simulink model "detection_algorithm_model"  (Simulink 7.7)
settings: Solver=VariableStepDiscrete  StartTime=0.0  StopTime=0.1  RelTol=1e-3
libraries: dsparch4 x1, dspstat3 x1, dspsrcs4 x1
settings Model: Creator=staticd  LastModifiedBy=staticd

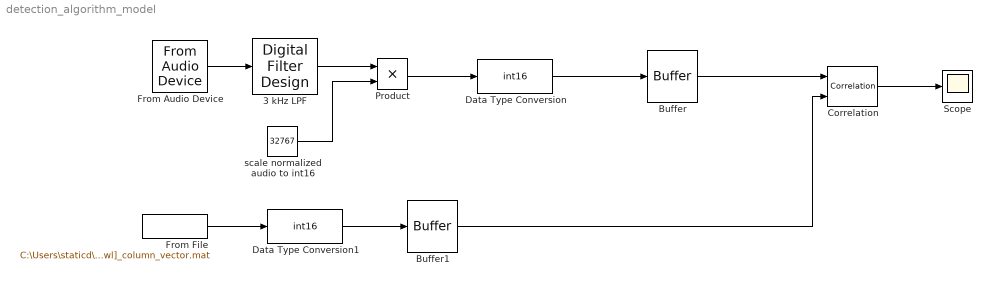
== system detection_algorithm_model ==
  3 kHz LPF : dsparch4/Digital Filter Design  SystemSampleTime=-1  mwdsp_browser_bugfix_var=off
  Buffer : Buffer  N=14000  TreatMby1Signals=One channel
  Buffer1 : Buffer  N=14000  TreatMby1Signals=One channel
  Correlation : dspstat3/Correlation  domain=Time  outputDataTypeStr=Inherit: Same as accumulator  outputLastDataTypeStr=Inherit: Same as accumulator  outputMin=[]  outputMax=[]  roundingMode=Floor  overflowMode=off
  Data Type Conversion : DataTypeConversion  OutDataTypeStr=int16
  Data Type Conversion1 : DataTypeConversion  OutDataTypeStr=int16
  From Audio Device : dspsrcs4/From Audio Device  deviceName=External Mic (IDT High Definition Audio CODEC)  numChannels=1  sampleRate=8e3  deviceDatatype=Determine from output data type  autoBufferSize=off  bufferSize=8172  queueDuration=1.0  frameSize=1024  outputDatatype=single
  From File : FromFile  FileName=C:\Users\staticd\Documents\My Dropbox\forLeo (2)\project\sample_data\soi_[growl]_column_vector.mat  SampleTime=8e3
  Product : Product  RndMeth=Zero
  Scope : Scope
  scale normalized audio to int16 : Constant  Value=32767  OutDataTypeStr=int16
  wires:
  From Audio Device/1 -> 3 kHz LPF/1
  3 kHz LPF/1 -> Product/1
  scale normalized audio to int16/1 -> Product/2
  Product/1 -> Data Type Conversion/1
  Data Type Conversion/1 -> Buffer/1
  From File/1 -> Data Type Conversion1/1
  Data Type Conversion1/1 -> Buffer1/1
  Buffer/1 -> Correlation/1
  Buffer1/1 -> Correlation/2
  Correlation/1 -> Scope/1
